simulink model "test2"  (R2018b)
settings: Solver=VariableStepAuto  StartTime=0.0  StopTime=10.0  RelTol=1e-3
settings Model: Creator=12732  LastModifiedBy=12732

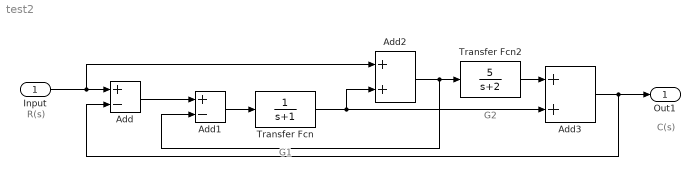
== system test2 ==
  note: G1
  note: G2
  note: C(s)
  note: R(s)
  Input : Inport
  Add : Sum  Inputs=+-
  Add1 : Sum  Inputs=+-
  Add2 : Sum
  Add3 : Sum
  Transfer Fcn : TransferFcn  Denominator=[1 1]
  Transfer Fcn2 : TransferFcn  Numerator=[5]  Denominator=[1 2]
  Out1 : Outport
  wires:
  Add1/1 -> Transfer Fcn/1
  Add/1 -> Add1/1
  Input/1 -> Add2/1, Add/1
  Transfer Fcn/1 -> Add3/2, Add2/2
  Add2/1 -> Add1/2, Transfer Fcn2/1
  Transfer Fcn2/1 -> Add3/1
  Add3/1 -> Out1/1, Add/2
